simulink model "DLQR_reference_tracking_simulink"  (R2023b)
settings: Solver=FixedStepAuto  StartTime=0.0  StopTime=60  FixedStep=1/1000  RelTol=1e-3
values from neighbouring files (symbols this model uses):
  h = 0.125    [Controllers_Design.m]    (also in DLMI_code_validation.m = 1; DLQR_rotational_controller_design.m = Pc_inv(end,:); DLQR_translational_controller.m = Pc_inv(end,:))
  m = 1220.24/1000    (= 1.22024)    [Controllers_Design.m]    (also in calculate_inclination_force.m; forceCompensationDueGlassInclination.m)
  tractor_max_force = 0.2238    [Controllers_Design.m]
  ts = 0.0521    [Controllers_Design.m]
undefined symbols (not defined in the file or in its folder): Gm, K_trans, tm
libraries: simulink_extras x2
settings Model: Creator=luanv  LastModifiedBy=Luan

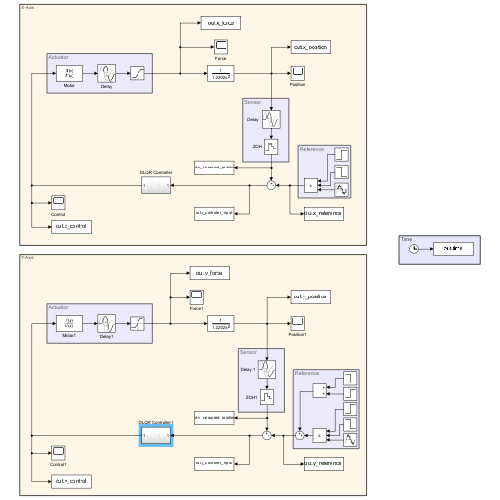
[thumbnail: Simulink's stored preview of the top-level diagram]
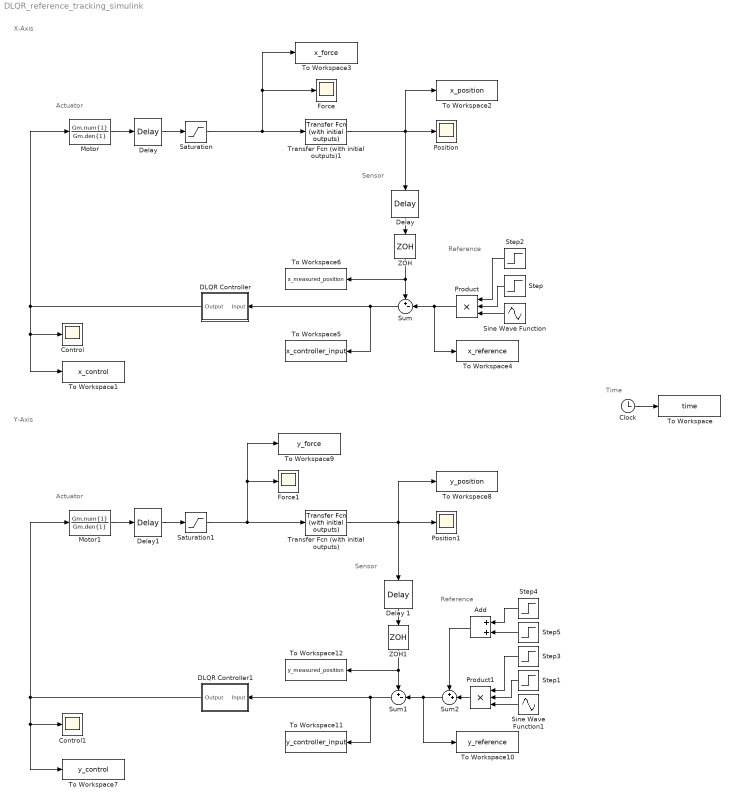
== system DLQR_reference_tracking_simulink ==
  note: Reference
  note: Reference
  note: Time
  note: X-Axis
  note: Sensor
  note: Actuator
  note: Sensor
  note: Y-Axis
  note: Actuator
  Add : Sum
  Clock : Clock
  Control : Scope
  Control1 : Scope
  DLQR Controller : Subsystem
  DLQR Controller1 : Subsystem
  Delay : TransportDelay  DelayTime=tm
  "Delay " : TransportDelay  DelayTime=ts
  Delay 1 : TransportDelay  DelayTime=ts  InitialOutput=0.3
  Delay1 : TransportDelay  DelayTime=tm
  Force : Scope
  Force1 : Scope
  Motor : TransferFcn  Numerator=Gm.num{1}  Denominator=Gm.den{1}
  Motor1 : TransferFcn  Numerator=Gm.num{1}  Denominator=Gm.den{1}
  Position : Scope
  Position1 : Scope
  Product : Product  Inputs=3
  Product1 : Product  Inputs=3
  Saturation : Saturate  UpperLimit=tractor_max_force  LowerLimit=-tractor_max_force
  Saturation1 : Saturate  UpperLimit=tractor_max_force  LowerLimit=-tractor_max_force
  Sine Wave Function : Sin  Amplitude=0.3  Frequency=(2*pi)/48  Phase=-(5*pi)/4  SampleTime=h
  Sine Wave Function1 : Sin  Amplitude=0.3  Frequency=(2*pi)/48  Phase=-(pi/4)+(pi/2)  SampleTime=h
  Step : Step  Time=54  Before=1  After=0  SampleTime=0
  Step1 : Step  Time=54  Before=1  After=0  SampleTime=0
  Step2 : Step  Time=6  SampleTime=0
  Step3 : Step  Time=6  SampleTime=0
  Step4 : Step  Time=6  Before=0.3  After=0  SampleTime=0
  Step5 : Step  Time=54  After=0.3  SampleTime=0
  Sum : Sum  Inputs=+-|
  Sum1 : Sum  Inputs=+-|
  Sum2 : Sum  Inputs=++|
  To Workspace : ToWorkspace  VariableName=time  SaveFormat=Timeseries  SampleTime=-1
  To Workspace1 : ToWorkspace  VariableName=x_control  SaveFormat=Timeseries  SampleTime=1/1000
  To Workspace10 : ToWorkspace  VariableName=y_reference  SaveFormat=Timeseries  SampleTime=1/1000
  To Workspace11 : ToWorkspace  VariableName=y_controller_input  SaveFormat=Timeseries  SampleTime=1/1000
  To Workspace12 : ToWorkspace  VariableName=y_measured_position  SaveFormat=Timeseries  SampleTime=1/1000
  To Workspace2 : ToWorkspace  VariableName=x_position  SaveFormat=Timeseries  SampleTime=-1
  To Workspace3 : ToWorkspace  VariableName=x_force  SaveFormat=Timeseries  SampleTime=-1
  To Workspace4 : ToWorkspace  VariableName=x_reference  SaveFormat=Timeseries  SampleTime=1/1000
  To Workspace5 : ToWorkspace  VariableName=x_controller_input  SaveFormat=Timeseries  SampleTime=1/1000
  To Workspace6 : ToWorkspace  VariableName=x_measured_position  SaveFormat=Timeseries  SampleTime=1/1000
  To Workspace7 : ToWorkspace  VariableName=y_control  SaveFormat=Timeseries  SampleTime=1/1000
  To Workspace8 : ToWorkspace  VariableName=y_position  SaveFormat=Timeseries  SampleTime=-1
  To Workspace9 : ToWorkspace  VariableName=y_force  SaveFormat=Timeseries  SampleTime=-1
  Transfer Fcn (with initial outputs) : simulink_extras/Additional Linear/Transfer Fcn (with initial outputs)  N=[1]  D=[m 0 0]  Y0=0.3  U0=0
  Transfer Fcn (with initial outputs)1 : simulink_extras/Additional Linear/Transfer Fcn (with initial outputs)  N=[1]  D=[m 0 0]  Y0=0  U0=0
  ZOH : ZeroOrderHold  SampleTime=h
  ZOH1 : ZeroOrderHold  SampleTime=h
  wires:
  Motor/1 -> Delay/1
  Transfer Fcn (with initial outputs)1/1 -> "Delay "/1, To Workspace2/1, Position/1
  Delay/1 -> Saturation/1
  Saturation/1 -> Transfer Fcn (with initial outputs)1/1, To Workspace3/1, Force/1
  DLQR Controller/1(Output) -> To Workspace1/1, Control/1, Motor/1
  Clock/1 -> To Workspace/1
  Sum/1 -> DLQR Controller/1(Input), To Workspace5/1
  Sum1/1 -> DLQR Controller1/1(Input), To Workspace11/1
  Delay1/1 -> Saturation1/1
  Saturation1/1 -> Transfer Fcn (with initial outputs)/1, To Workspace9/1, Force1/1
  DLQR Controller1/1(Output) -> To Workspace7/1, Control1/1, Motor1/1
  Motor1/1 -> Delay1/1
  Sine Wave Function/1 -> Product/3
  Step/1 -> Product/2
  Step2/1 -> Product/1
  Sine Wave Function1/1 -> Product1/3
  Step3/1 -> Product1/1
  Step1/1 -> Product1/2
  Step5/1 -> Add/2
  Product1/1 -> Sum2/2
  Sum2/1 -> To Workspace10/1, Sum1/2
  Step4/1 -> Add/1
  Add/1 -> Sum2/1
  "Delay "/1 -> ZOH/1
  ZOH/1 -> To Workspace6/1, Sum/1
  Delay 1/1 -> ZOH1/1
  ZOH1/1 -> To Workspace12/1, Sum1/1
  Transfer Fcn (with initial outputs)/1 -> To Workspace8/1, Position1/1, Delay 1/1
  Product/1 -> Sum/2, To Workspace4/1

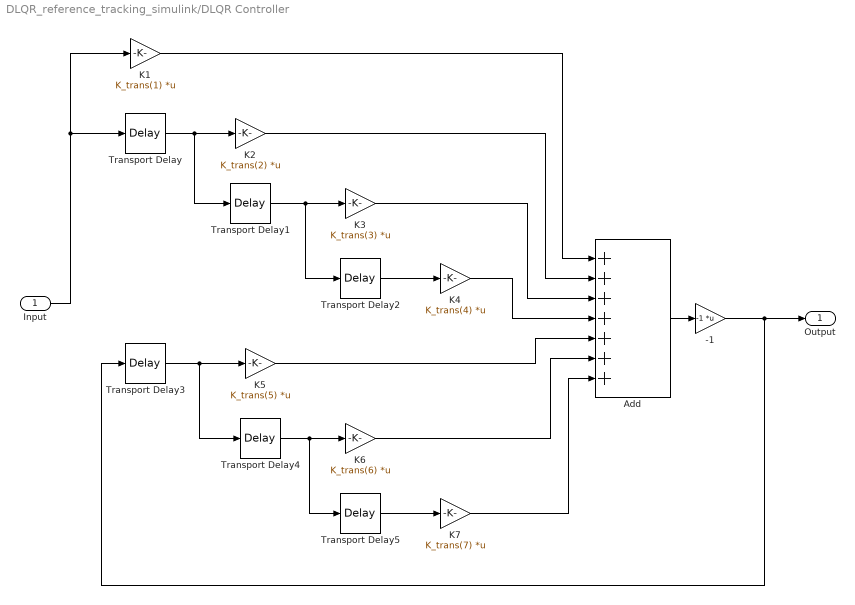
== system DLQR_reference_tracking_simulink/DLQR Controller ==
  Input : Inport
  -1 : Gain  Gain=-1  Multiplication=Matrix(K*u)
  Add : Sum  Inputs=+++++++
  K1 : Gain  Gain=K_trans(1)  Multiplication=Matrix(K*u)
  K2 : Gain  Gain=K_trans(2)  Multiplication=Matrix(K*u)
  K3 : Gain  Gain=K_trans(3)  Multiplication=Matrix(K*u)
  K4 : Gain  Gain=K_trans(4)  Multiplication=Matrix(K*u)
  K5 : Gain  Gain=K_trans(5)  Multiplication=Matrix(K*u)
  K6 : Gain  Gain=K_trans(6)  Multiplication=Matrix(K*u)
  K7 : Gain  Gain=K_trans(7)  Multiplication=Matrix(K*u)
  Transport Delay{,1..5} (6 alike) : TransportDelay  DelayTime=h
  Output : Outport
  wires:
  Input/1 -> Transport Delay/1, K1/1
  Transport Delay/1 -> Transport Delay1/1, K2/1
  Transport Delay1/1 -> Transport Delay2/1, K3/1
  Transport Delay2/1 -> K4/1
  Transport Delay3/1 -> Transport Delay4/1, K5/1
  Transport Delay4/1 -> Transport Delay5/1, K6/1
  Transport Delay5/1 -> K7/1
  K1/1 -> Add/1
  K2/1 -> Add/2
  K3/1 -> Add/3
  K4/1 -> Add/4
  K5/1 -> Add/5
  K6/1 -> Add/6
  K7/1 -> Add/7
  Add/1 -> -1/1
  -1/1 -> Transport Delay3/1, Output/1

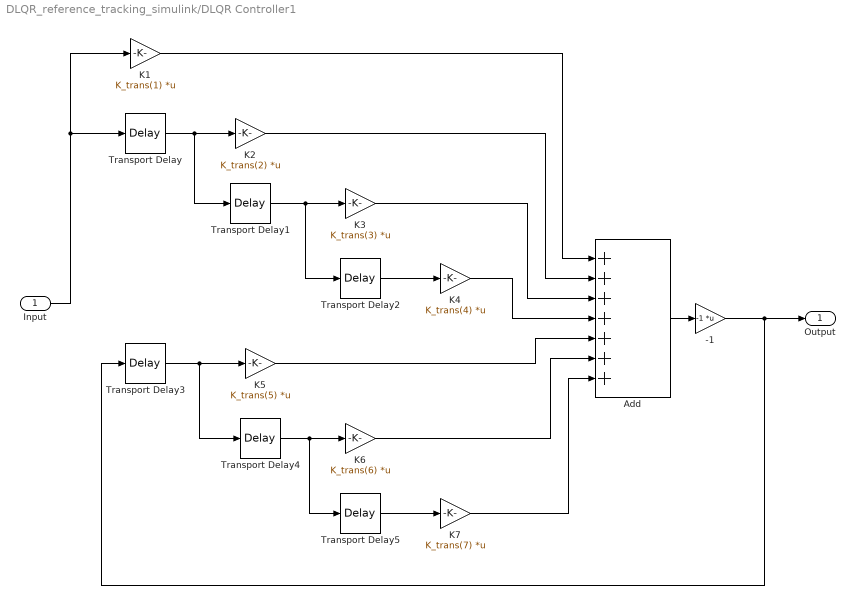
== system DLQR_reference_tracking_simulink/DLQR Controller1 ==
  Input : Inport
  -1 : Gain  Gain=-1  Multiplication=Matrix(K*u)
  Add : Sum  Inputs=+++++++
  K1 : Gain  Gain=K_trans(1)  Multiplication=Matrix(K*u)
  K2 : Gain  Gain=K_trans(2)  Multiplication=Matrix(K*u)
  K3 : Gain  Gain=K_trans(3)  Multiplication=Matrix(K*u)
  K4 : Gain  Gain=K_trans(4)  Multiplication=Matrix(K*u)
  K5 : Gain  Gain=K_trans(5)  Multiplication=Matrix(K*u)
  K6 : Gain  Gain=K_trans(6)  Multiplication=Matrix(K*u)
  K7 : Gain  Gain=K_trans(7)  Multiplication=Matrix(K*u)
  Transport Delay{,1..5} (6 alike) : TransportDelay  DelayTime=h
  Output : Outport
  wires:
  Input/1 -> Transport Delay/1, K1/1
  Transport Delay/1 -> Transport Delay1/1, K2/1
  Transport Delay1/1 -> Transport Delay2/1, K3/1
  Transport Delay2/1 -> K4/1
  Transport Delay3/1 -> Transport Delay4/1, K5/1
  Transport Delay4/1 -> Transport Delay5/1, K6/1
  Transport Delay5/1 -> K7/1
  K1/1 -> Add/1
  K2/1 -> Add/2
  K3/1 -> Add/3
  K4/1 -> Add/4
  K5/1 -> Add/5
  K6/1 -> Add/6
  K7/1 -> Add/7
  Add/1 -> -1/1
  -1/1 -> Transport Delay3/1, Output/1
